simulink model "AV9_5"  (R2018a)
settings: Solver=VariableStepAuto  StartTime=0.0  StopTime=100  RelTol=1e-3
values from neighbouring files (symbols this model uses):
  q0 = -1.1901    [AV10_ZADACHA1.m]    (also in AV9_PRIMER2_VREDNOSTI.m = -62.3782; AV9_PRIMER4.m = 1.9573; AV9_PRIMER5.m = 1.8649; AV_10_PRIMER1.m = 1.512)
  q1 = 0.8945    [AV10_ZADACHA1.m]    (also in AV9_PRIMER2_VREDNOSTI.m = 122.0694; AV9_PRIMER4.m = -1.6594; AV9_PRIMER5.m = -1.8649; AV_10_PRIMER1.m = -1.423)
  q2 = -0.2805    [AV10_ZADACHA1.m]    (also in AV9_PRIMER2_VREDNOSTI.m = -59.9743; AV9_PRIMER4.m = 0.6675; AV9_PRIMER5.m = 0.2403; AV_10_PRIMER1.m = 0.44)
  T = 160    [AV10_ZADACHA1.m]    (also in AV9_PRIMER4.m = 16; AV9_PRIMER5.m = 4; AV_10_PRIMER1.m = 8)
settings Model: Creator=DD  LastModifiedBy=DD

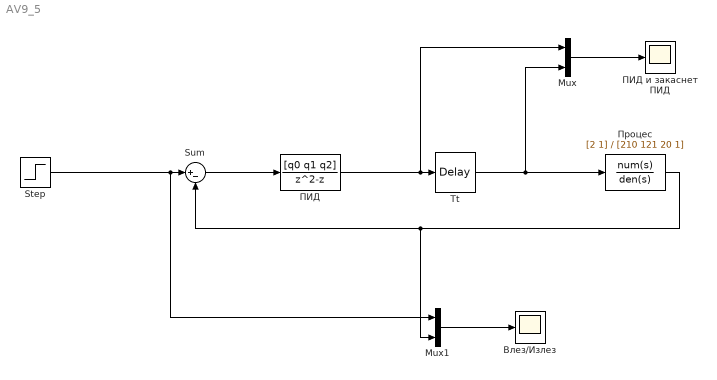
== system AV9_5 ==
  Mux : Mux  Inputs=2
  Mux1 : Mux  Inputs=2
  Step : Step  Before=1  SampleTime=0
  Sum : Sum  Inputs=|+-
  "Влез/Излез " : Scope
  "ПИД " : DiscreteTransferFcn  Numerator=[q0 q1 q2]  Denominator=[1 -1 0]  SampleTime=T
  ПИД и закаснет ПИД : Scope
  "Процес " : TransferFcn  Numerator=[2 1]  Denominator=[210 121 20 1]
  Тt : TransportDelay  DelayTime=4
  wires:
  Step/1 -> Mux1/1, Sum/1
  Sum/1 -> "ПИД "/1
  "ПИД "/1 -> Mux/1, Тt/1
  Тt/1 -> Mux/2, "Процес "/1
  Mux/1 -> ПИД и закаснет ПИД/1
  "Процес "/1 -> Mux1/2, Sum/2
  Mux1/1 -> "Влез/Излез "/1
